simulink model "xt2_2"  (R2014a)
settings: Solver=ode45  StartTime=0.0  StopTime=20  MaxStep=0.1  RelTol=1e-3
libraries: simulink x1
settings Model: Creator=tzb  LastModifiedBy=tzb

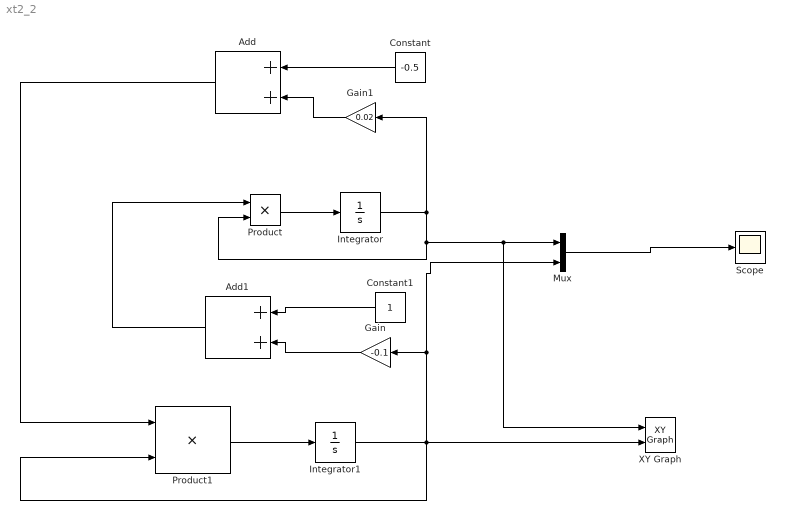
== system xt2_2 ==
  Add : Sum
  Add1 : Sum
  Constant : Constant  Value=-0.5
  Constant1 : Constant
  Gain : Gain  Gain=-0.1
  Gain1 : Gain  Gain=0.02
  Integrator : Integrator  InitialCondition=25
  Integrator1 : Integrator  InitialCondition=2
  Mux : Mux  Inputs=2
  Product : Product
  Product1 : Product
  Scope : Scope
  XY Graph : simulink/Sinks/XY Graph  xmin=0  xmax=120  ymin=0  ymax=120  st=-1
  wires:
  Constant/1 -> Add/1
  Product/1 -> Integrator/1
  Add/1 -> Product1/1
  Product1/1 -> Integrator1/1
  Gain/1 -> Add1/2
  Integrator1/1 -> XY Graph/2, Mux/2, Gain/1, Product1/2
  Add1/1 -> Product/1
  Constant1/1 -> Add1/1
  Gain1/1 -> Add/2
  Integrator/1 -> XY Graph/1, Mux/1, Product/2, Gain1/1
  Mux/1 -> Scope/1
